simulink model "planLocalPath"  (R2024a)
settings: Solver=FixedStepDiscrete  StartTime=0.0  StopTime=10.0  RelTol=1e-3
undefined symbols (not defined in the file or in its folder): fixedTEBParams, maxLocalPathLen, maxRefPathLen
settings Model: Creator=cstabile  LastModifiedBy=cstabile
settings SFSimCC: SimTargetLang=C++

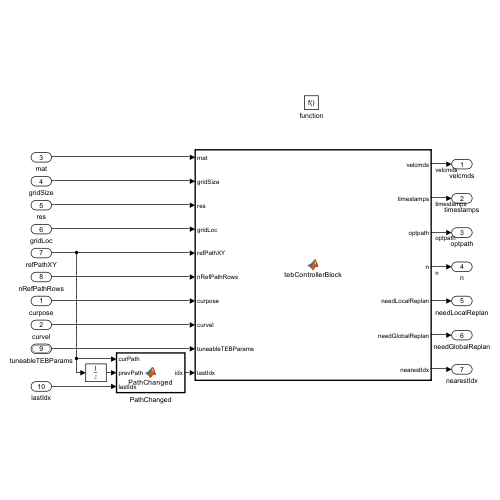
[thumbnail: Simulink's stored preview of the top-level diagram]
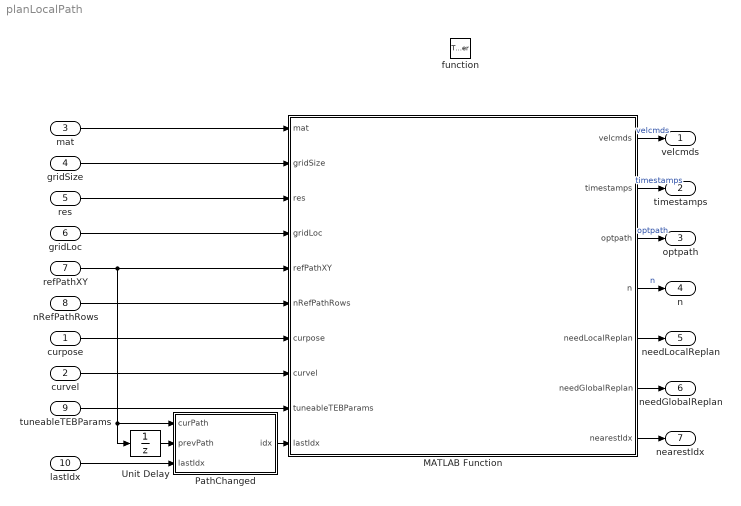
== system planLocalPath ==
  curpose : Inport
  curvel : Inport  Port=2
  mat : Inport  Port=3  OutDataTypeStr=boolean  PortDimensions=[1201 1201]  Interpolate=off
      settings: VarSizeSig=Yes
  gridSize : Inport  Port=4
  res : Inport  Port=5
  gridLoc : Inport  Port=6
  refPathXY : Inport  Port=7  PortDimensions=[maxRefPathLen 3]  Interpolate=off
  nRefPathRows : Inport  Port=8
  tuneableTEBParams : Inport  Port=9  OutDataTypeStr=Bus: teb_bus
  lastIdx : Inport  Port=10
  function : TriggerPort  TriggerType=function-call  VariantControl=(inherit)
  MATLAB Function : MATLAB Function  TreatAsAtomicUnit=on  mask{length=fixedTEBParams.Length, width=fixedTEBParams.Width, numIteration=fixedTEBParams.NumIteration, referenceDeltaTime=fixedTEBParams.ReferenceDeltaTime, nRowOutput=maxLocalPathLen}
      mask prompts: length "Length of vehicle (in meters)"; width "Width of vehicle (in meters)"; numIteration "Number of optimization iterations per call"; referenceDeltaTime "Desired timespan between control commands (in seconds)"; nRowOutput "MaxNumOutput"
  PathChanged : MATLAB Function  TreatAsAtomicUnit=on
  Unit Delay : UnitDelay  SampleTime=-1  HasFrameUpgradeWarning=on
  velcmds : Outport  OutDataTypeStr=double  PortDimensions=[1000 2]
  timestamps : Outport  Port=2  OutDataTypeStr=double  PortDimensions=[1000 1]
  optpath : Outport  Port=3  OutDataTypeStr=double  PortDimensions=[1000 3]
  n : Outport  Port=4  OutDataTypeStr=double  PortDimensions=1
  needLocalReplan : Outport  Port=5  OutDataTypeStr=double  PortDimensions=1
  needGlobalReplan : Outport  Port=6  OutDataTypeStr=double  PortDimensions=1
  nearestIdx : Outport  Port=7
  wires:
  gridSize/1 -> MATLAB Function/2(gridSize)
  curpose/1 -> MATLAB Function/7(curpose)
  tuneableTEBParams/1 -> MATLAB Function/9(tuneableTEBParams)
  curvel/1 -> MATLAB Function/8(curvel)
  refPathXY/1 -> MATLAB Function/5(refPathXY), Unit Delay/1, PathChanged/1(curPath)
  mat/1 -> MATLAB Function/1(mat)
  nRefPathRows/1 -> MATLAB Function/6(nRefPathRows)
  gridLoc/1 -> MATLAB Function/4(gridLoc)
  MATLAB Function/3(optpath) -> optpath/1  "optpath"
  MATLAB Function/6(needGlobalReplan) -> needGlobalReplan/1
  MATLAB Function/4(n) -> n/1  "n"
  MATLAB Function/5(needLocalReplan) -> needLocalReplan/1
  MATLAB Function/1(velcmds) -> velcmds/1  "velcmds"
  MATLAB Function/2(timestamps) -> timestamps/1  "timestamps"
  res/1 -> MATLAB Function/3(res)
  MATLAB Function/7(nearestIdx) -> nearestIdx/1
  Unit Delay/1 -> PathChanged/2(prevPath)
  PathChanged/1(idx) -> MATLAB Function/10(lastIdx)
  lastIdx/1 -> PathChanged/3(lastIdx)

== matlab function planLocalPath/PathChanged ==
  data: curPath input; prevPath input; lastIdx input; idx output
function idx = PathChanged(curPath, prevPath, lastIdx)
%PathChanged Reset the nearest index when new path has been provided
    if ~isequal(curPath,prevPath)
        idx = 1;
    else
        idx = lastIdx;
    end
end

== matlab function planLocalPath/MATLAB Function ==
  data: mat input; gridSize input size=[1 2]; res input; velcmds output size=[nRowOutput 2]; gridLoc input size=[1 2]; refPathXY input size=[maxRefPathLen 3]; nRefPathRows input; curpose input size=[1 3]; curvel input size=[1 2]; tuneableTEBParams input Bus: teb_bus; timestamps output size=[nRowOutput 1]; optpath output size=[nRowOutput 3]; length parameter; width parameter; numIteration parameter; referenceDeltaTime parameter; n output size=[1 1]; nRowOutput parameter; needLocalReplan output; needGlobalReplan output; lastIdx input; nearestIdx output
function [velcmds,timestamps,optpath,n,needLocalReplan,needGlobalReplan,nearestIdx] = tebControllerBlock(mat, gridSize, res, ...
    gridLoc, refPathXY, nRefPathRows, curpose, curvel, tuneableTEBParams, ...
    length, width, numIteration, referenceDeltaTime, nRowOutput, lastIdx)
    
    velcmds = nan(nRowOutput,2);
    timestamps = nan(nRowOutput,1);
    optpath = nan(nRowOutput,3);
    n = 0;
    needLocalReplan = 0;
    needGlobalReplan = 0;
    nearestIdx = 1;
    if nRefPathRows ~= 0
        egoMat = mat(1:gridSize(1),1:gridSize(2));

        [velcmds_,timestamps_,optpath_,nearestIdx,info,needLocalReplan,needGlobalReplan] = TEBControllerFcn(egoMat, res, gridLoc, ...
            refPathXY(1:nRefPathRows,:), lastIdx, curpose, curvel, tuneableTEBParams, ...
            length, width, numIteration, referenceDeltaTime);

        n = numel(timestamps_);
        velcmds(1:n,:)      = velcmds_;
        timestamps(1:n,:)   = timestamps_;
        optpath(1:n,:)      = optpath_;
    end
end
